simulink model "blance_robot"  (R2024a)
settings: Solver=VariableStepAuto  StartTime=0.0  StopTime=20  RelTol=1e-3
values from neighbouring files (symbols this model uses):
  K_cons = [-4.92635870386 -6.18040077772 -1.81074270733 -1.19207999822 -32.1009473092 -3.5760389828 4.18688097447 0.16514939939 0.944125254207 0.571537384386 -4.92635870394 -6.18040077751 ... (240 elements, 40x6)]    [K_cons.mat]    (also in k_calc.m = zeros(40,6))
  X = [x1, x2, x1sq, x2sq, x1x2]    [k_calc.m]
undefined symbols (not defined in the file or in its folder): Y, Z
libraries: sm_lib x58, nesl_utility x18, slpidlib x2
(part 1 of 3)
settings Model: Creator=zhuho  LastModifiedBy=zhuho

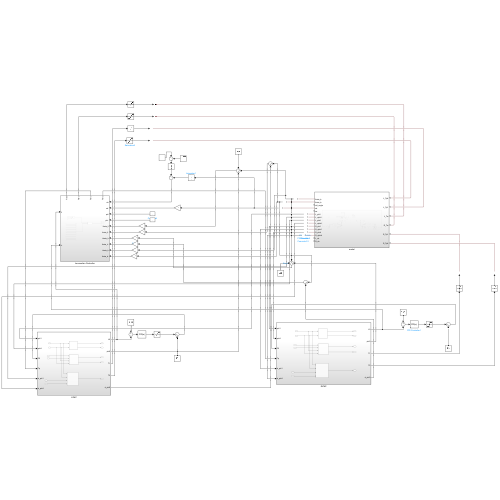
[thumbnail: Simulink's stored preview of the top-level diagram]
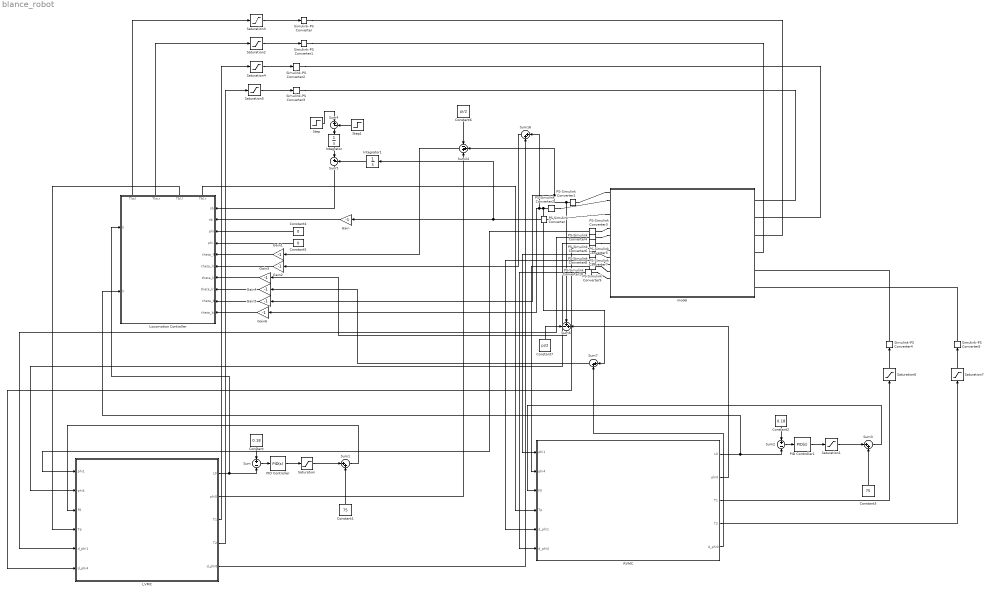
== system blance_robot ==
  Constant : Constant  Value=0.18
  Constant1 : Constant  Value=75
  Constant2 : Constant  Value=0.18
  Constant3 : Constant  Value=75
  Constant4 : Constant  Value=0
  Constant5 : Constant  Value=0
  Constant6 : Constant  Value=pi/2
  Constant7 : Constant  Value=pi/2
  Gain{,1..6} (7 alike) : Gain  Gain=-1
  Integrator : Integrator
  Integrator1 : Integrator
  LVMC : Subsystem
  Locomotion Controller : Subsystem
      settings: PortSchema="{\"entries\":[{\"content\":{\"sides\":[{\"content\":{\"connectorIds\":[\"In1\",\"In2\"]},\"type\":\"ConnectorPlacement.EquallySpacedRectSide\",\"uuid\":\"9f335f1a-920c-489c-ab23-b2605db4f7eb\"},{\"content\":{\"connectorIds\":[\"In3\",\"In4\",\"In5\",\"In6\",\"In7\",\"In8\",\"In9\",\"In10\",\"In11\",\"In12\"],\"side\":\"RIGHT\"},\"type\":\"ConnectorPlacement.EquallySpacedRectSide\",\"uuid\":\"244eb674-a427-495d-a4b5-69ad08e1900d\"},{\"content\":{\"connectorIds\":[\"Out1\",\"Out2\",\"Out3\",\"Out4\"],\"side\":\"TOP\"},\"type\":\"ConnectorPlacement.EquallySpacedRectSide\",\"uuid\":\"a2322f66-0ec6-4fc3-82d4-b6858da1a4af\"}]},\"type\":\"ConnectorPlacement.EquallySpacedConnector\",\"uuid\":\"7ddcb355-7f50-43e9-8496-f4eccb1abc77\"}],\"packageUris\":[\"http://schema.mathworks.com/mf0/Connector/R2020b\"],\"version\":\"1.0\"}"
  PID Controller : slpidlib/PID Controller  Controller=PID  Form=Parallel  TimeDomain=Continuous-time  UseExternalTs=off  SampleTime=-1  IntegratorMethod=Forward Euler  FilterMethod=Forward Euler  ControllerParametersSource=internal  P=500  I=0  UseKiTs=off  D=200  UseExternalDerivativeSource=off  N=100  UseFilter=on  TunerSelectOption=Transfer Function Based (PID Tuner App)  InitialConditionSource=internal  InitialConditionForIntegrator=0  InitialConditionForFilter=0  DifferentiatorICPrevScaledInput=0  ExternalReset=none  TrackingMode=off  Kt=1  LimitOutput=off  SatLimitsSource=internal  UpperSaturationLimit=inf  LowerSaturationLimit=-inf  LinearizeAsGain=on  AntiWindupMode=none  Kb=1  LimitIntegrator=off  UpperIntegratorSaturationLimit=inf  LowerIntegratorSaturationLimit=-inf  POutMin=[]  POutMax=[]  IOutMin=[]  IOutMax=[]  DOutMin=[]  DOutMax=[]  NOutMin=[]  NOutMax=[]  SumOutMin=[]  SumOutMax=[]  SaturationOutMin=[]  SaturationOutMax=[]  PParamMin=[]  PParamMax=[]  IParamMin=[]  IParamMax=[]  DParamMin=[]  DParamMax=[]  NParamMin=[]  NParamMax=[]  KbParamMin=[]  KbParamMax=[]  KtParamMin=[]  KtParamMax=[]  KbOutMin=[]  KbOutMax=[]  KtOutMin=[]  KtOutMax=[]  IntegratorOutMin=[]  IntegratorOutMax=[]  FilterOutMin=[]  FilterOutMax=[]  SumI1OutMin=[]  SumI1OutMax=[]  SumI2OutMin=[]  SumI2OutMax=[]  SumI3OutMin=[]  SumI3OutMax=[]  SumI4OutMin=[]  SumI4OutMax=[]  SumDOutMin=[]  SumDOutMax=[]  DifferentiatorOutMin=[]  DifferentiatorOutMax=[]  FilterDiffOutCoefMin=[]  FilterDiffOutCoefMax=[]  ReciprocalOutMin=[]  ReciprocalOutMax=[]  SumDenOutMin=[]  SumDenOutMax=[]  SumNumOutMin=[]  SumNumOutMax=[]  DivideOutMin=[]  DivideOutMax=[]  UdiffTsProdOutMin=[]  UdiffTsProdOutMax=[]  NTsProdOutMin=[]  NTsProdOutMax=[]  UintegralTsProdOutMin=[]  UintegralTsProdOutMax=[]  UngainTsProdOutMin=[]  UngainTsProdOutMax=[]  ClampingZeroOutDataTypeStr=Inherit: Inherit via back propagation  ClampingZeroOutMin=[]  ClampingZeroOutMax=[]  FilterDenConstantOutDataTypeStr=Inherit: Inherit via back propagation  FilterDenConstantOutMin=[]  FilterDenConstantOutMax=[]  PCopyOutDataTypeStr=Inherit: Inherit via back propagation  PCopyOutMin=[]  PCopyOutMax=[]  NCopyOutDataTypeStr=Inherit: Inherit via back propagation  NCopyOutMin=[]  NCopyOutMax=[]  IntegratorContinuousStateAttributes=''  IntegratorStateMustResolveToSignalObject=off  IntegratorRTWStateStorageClass=Auto  FilterContinuousStateAttributes=''  FilterStateMustResolveToSignalObject=off  FilterRTWStateStorageClass=Auto  ParallelPVariant=InternalParameters  IdealPVariant=Disabled  IVariant=InternalParameters  DVariant=InternalParameters  IntegratorVariant=Continuous  SatVariant=Disabled  AWVariant=Passthrough  PCopyVariant=Disabled  TRVariant=Disabled  FdbkBlocksVariant=Forward  IdealPFdbkVariant=Disabled  SatFdbkVariant=Disabled  DerivativeFilterVariant=ContFilter  NVariant=InternalParameters  NCopyVariant=Disabled  FilterICVariant=InternalICsFilter  IntegratorICVariant=InternalICs  ExternalResetVariant=Disabled  TRSumVariant=Passthrough  SumFdbkVariant=Disabled  SumVariant=Sum_PID  TsampFilterVariant=InternalTs  TsampNgainVariant=Passthrough  TsampIntegralVariant=Disabled_SignalSpec  ExternalSaturationOutDataTypeStr=Inherit: Same as second input  DerivativeSourceVariant=ErrorSignal
  PID Controller1 : slpidlib/PID Controller  Controller=PID  Form=Parallel  TimeDomain=Continuous-time  UseExternalTs=off  SampleTime=-1  IntegratorMethod=Forward Euler  FilterMethod=Forward Euler  ControllerParametersSource=internal  P=500  I=0  UseKiTs=off  D=200  UseExternalDerivativeSource=off  N=100  UseFilter=on  TunerSelectOption=Transfer Function Based (PID Tuner App)  InitialConditionSource=internal  InitialConditionForIntegrator=0  InitialConditionForFilter=0  DifferentiatorICPrevScaledInput=0  ExternalReset=none  TrackingMode=off  Kt=1  LimitOutput=off  SatLimitsSource=internal  UpperSaturationLimit=inf  LowerSaturationLimit=-inf  LinearizeAsGain=on  AntiWindupMode=none  Kb=1  LimitIntegrator=off  UpperIntegratorSaturationLimit=inf  LowerIntegratorSaturationLimit=-inf  POutMin=[]  POutMax=[]  IOutMin=[]  IOutMax=[]  DOutMin=[]  DOutMax=[]  NOutMin=[]  NOutMax=[]  SumOutMin=[]  SumOutMax=[]  SaturationOutMin=[]  SaturationOutMax=[]  PParamMin=[]  PParamMax=[]  IParamMin=[]  IParamMax=[]  DParamMin=[]  DParamMax=[]  NParamMin=[]  NParamMax=[]  KbParamMin=[]  KbParamMax=[]  KtParamMin=[]  KtParamMax=[]  KbOutMin=[]  KbOutMax=[]  KtOutMin=[]  KtOutMax=[]  IntegratorOutMin=[]  IntegratorOutMax=[]  FilterOutMin=[]  FilterOutMax=[]  SumI1OutMin=[]  SumI1OutMax=[]  SumI2OutMin=[]  SumI2OutMax=[]  SumI3OutMin=[]  SumI3OutMax=[]  SumI4OutMin=[]  SumI4OutMax=[]  SumDOutMin=[]  SumDOutMax=[]  DifferentiatorOutMin=[]  DifferentiatorOutMax=[]  FilterDiffOutCoefMin=[]  FilterDiffOutCoefMax=[]  ReciprocalOutMin=[]  ReciprocalOutMax=[]  SumDenOutMin=[]  SumDenOutMax=[]  SumNumOutMin=[]  SumNumOutMax=[]  DivideOutMin=[]  DivideOutMax=[]  UdiffTsProdOutMin=[]  UdiffTsProdOutMax=[]  NTsProdOutMin=[]  NTsProdOutMax=[]  UintegralTsProdOutMin=[]  UintegralTsProdOutMax=[]  UngainTsProdOutMin=[]  UngainTsProdOutMax=[]  ClampingZeroOutDataTypeStr=Inherit: Inherit via back propagation  ClampingZeroOutMin=[]  ClampingZeroOutMax=[]  FilterDenConstantOutDataTypeStr=Inherit: Inherit via back propagation  FilterDenConstantOutMin=[]  FilterDenConstantOutMax=[]  PCopyOutDataTypeStr=Inherit: Inherit via back propagation  PCopyOutMin=[]  PCopyOutMax=[]  NCopyOutDataTypeStr=Inherit: Inherit via back propagation  NCopyOutMin=[]  NCopyOutMax=[]  IntegratorContinuousStateAttributes=''  IntegratorStateMustResolveToSignalObject=off  IntegratorRTWStateStorageClass=Auto  FilterContinuousStateAttributes=''  FilterStateMustResolveToSignalObject=off  FilterRTWStateStorageClass=Auto  ParallelPVariant=InternalParameters  IdealPVariant=Disabled  IVariant=InternalParameters  DVariant=InternalParameters  IntegratorVariant=Continuous  SatVariant=Disabled  AWVariant=Passthrough  PCopyVariant=Disabled  TRVariant=Disabled  FdbkBlocksVariant=Forward  IdealPFdbkVariant=Disabled  SatFdbkVariant=Disabled  DerivativeFilterVariant=ContFilter  NVariant=InternalParameters  NCopyVariant=Disabled  FilterICVariant=InternalICsFilter  IntegratorICVariant=InternalICs  ExternalResetVariant=Disabled  TRSumVariant=Passthrough  SumFdbkVariant=Disabled  SumVariant=Sum_PID  TsampFilterVariant=InternalTs  TsampNgainVariant=Passthrough  TsampIntegralVariant=Disabled_SignalSpec  ExternalSaturationOutDataTypeStr=Inherit: Same as second input  DerivativeSourceVariant=ErrorSignal
  PS-Simulink Converter{,1..10} (11 alike) : nesl_utility/PS-Simulink Converter  PhysicalDomain=network_engine_domain  SubClassName=ps_output  LeftPortType=input  RightPortType=output  PseudoPeriodic=off  Frequencies=[]  VectorFormat=inherit  Unit=inherit  AffineConversion=off
  RVMC : Subsystem
  Saturation : Saturate  UpperLimit=9  LowerLimit=-9
  Saturation1 : Saturate  UpperLimit=9  LowerLimit=-9
  Saturation{2..7} (6 alike) : Saturate  UpperLimit=10  LowerLimit=-10
  Simulink-PS Converter{,1..5} (6 alike) : nesl_utility/Simulink-PS Converter  PhysicalDomain=network_engine_domain  SubClassName=ps_input  LeftPortType=input  RightPortType=output  PseudoPeriodic=off  Frequencies=[]  NoiseDistribution=none  NoiseParameters=[]  Unit=1  AffineConversion=off  FilteringAndDerivatives=provide  SimscapeFilterOrder=1  InputFilterTimeConstant=0.001  UdotUserProvided=0
  Step : Step  Time=0.8  After=2.5  SampleTime=0
  Step1 : Step  Time=5  After=2.5  SampleTime=0
  Sum : Sum  Inputs=+|-
  Sum{1,3,7,16} (4 alike) : Sum  Inputs=|++
  Sum2 : Sum  Inputs=+|-
  Sum24 : Sum  Inputs=-++
  Sum4 : Sum  Inputs=|+-
  Sum5 : Sum  Inputs=|+-
  Sum6 : Sum  Inputs=-++
  model : Subsystem
  wires:
  Constant/1 -> Sum/1
  Sum/1 -> PID Controller/1
  PID Controller/1 -> Saturation/1
  Constant1/1 -> Sum1/2
  Saturation/1 -> Sum1/1
  Sum1/1 -> LVMC/3(F0)
  Locomotion Controller/3(Tbl,l) -> LVMC/4(Tp)
  Locomotion Controller/4(Tbl,r) -> RVMC/4(Tp)
  Constant2/1 -> Sum2/1
  Sum2/1 -> PID Controller1/1
  PID Controller1/1 -> Saturation1/1
  Constant3/1 -> Sum3/2
  Saturation1/1 -> Sum3/1
  Sum3/1 -> RVMC/3(F0)
  LVMC/1(L0) -> Locomotion Controller/1(ll), Sum/2
  RVMC/1(L0) -> Locomotion Controller/2(lr), Sum2/2
  Locomotion Controller/1(Tlw,l) -> Saturation3/1
  Locomotion Controller/2(Tlw,r) -> Saturation2/1
  Saturation2/1 -> Simulink-PS Converter1/1
  Saturation3/1 -> Simulink-PS Converter/1
  LVMC/4(T2) -> Saturation5/1
  LVMC/3(T1) -> Saturation4/1
  Saturation4/1 -> Simulink-PS Converter2/1
  Saturation5/1 -> Simulink-PS Converter3/1
  RVMC/3(T1) -> Saturation6/1
  Saturation6/1 -> Simulink-PS Converter4/1
  RVMC/4(T2) -> Saturation7/1
  Saturation7/1 -> Simulink-PS Converter5/1
  PS-Simulink Converter/1 -> Integrator1/1, Gain/1
  Gain/1 -> Locomotion Controller/4(sb.)
  Step/1 -> Sum4/1
  Step1/1 -> Sum4/2
  Sum4/1 -> Integrator/1
  Integrator/1 -> Sum5/1
  Sum5/1 -> Locomotion Controller/3(sb)
  Integrator1/1 -> Sum5/2
  Constant4/1 -> Locomotion Controller/5(phi)
  Constant5/1 -> Locomotion Controller/6(phi.)
  Constant6/1 -> Sum24/1
  Sum24/1 -> Gain1/1
  LVMC/2(phi0) -> Sum24/3
  PS-Simulink Converter1/1 -> Gain5/1, Sum24/2, Sum6/2
  Gain1/1 -> Locomotion Controller/7(theta_ll)
  PS-Simulink Converter2/1 -> Sum7/1, Gain6/1, Sum16/1
  LVMC/5(d_phi0) -> Sum16/2
  Sum16/1 -> Gain2/1
  Gain2/1 -> Locomotion Controller/8(theta_ll.)
  Constant7/1 -> Sum6/1
  RVMC/2(phi0) -> Sum6/3
  Sum6/1 -> Gain3/1
  RVMC/5(d_phi0) -> Sum7/2
  Sum7/1 -> Gain4/1
  Gain3/1 -> Locomotion Controller/9(theta_lr)
  Gain4/1 -> Locomotion Controller/10(theta_lr.)
  Gain5/1 -> Locomotion Controller/11(theta_b)
  Gain6/1 -> Locomotion Controller/12(theta_b.)
  PS-Simulink Converter3/1 -> LVMC/1(phi1)
  PS-Simulink Converter4/1 -> LVMC/5(d_phi1)
  PS-Simulink Converter5/1 -> LVMC/2(phi4)
  PS-Simulink Converter6/1 -> LVMC/6(d_phi4)
  PS-Simulink Converter7/1 -> RVMC/1(phi1)
  PS-Simulink Converter9/1 -> RVMC/2(phi4)
  PS-Simulink Converter8/1 -> RVMC/5(d_phi1)
  PS-Simulink Converter10/1 -> RVMC/6(d_phi4)
  connections:
  model/RConn4 -- PS-Simulink Converter/LConn1
  Simulink-PS Converter/RConn1 -- model/LConn3
  Simulink-PS Converter1/RConn1 -- model/LConn4
  Simulink-PS Converter2/RConn1 -- model/LConn2
  Simulink-PS Converter3/RConn1 -- model/LConn1
  Simulink-PS Converter4/RConn1 -- model/LConn5
  Simulink-PS Converter5/RConn1 -- model/LConn6
  model/RConn1 -- PS-Simulink Converter1/LConn1
  PS-Simulink Converter2/LConn1 -- model/RConn2
  PS-Simulink Converter3/LConn1 -- model/RConn6
  PS-Simulink Converter4/LConn1 -- model/RConn7
  PS-Simulink Converter5/LConn1 -- model/RConn8
  PS-Simulink Converter6/LConn1 -- model/RConn9
  PS-Simulink Converter7/LConn1 -- model/RConn10
  PS-Simulink Converter8/LConn1 -- model/RConn11
  PS-Simulink Converter9/LConn1 -- model/RConn12
  PS-Simulink Converter10/LConn1 -- model/RConn13

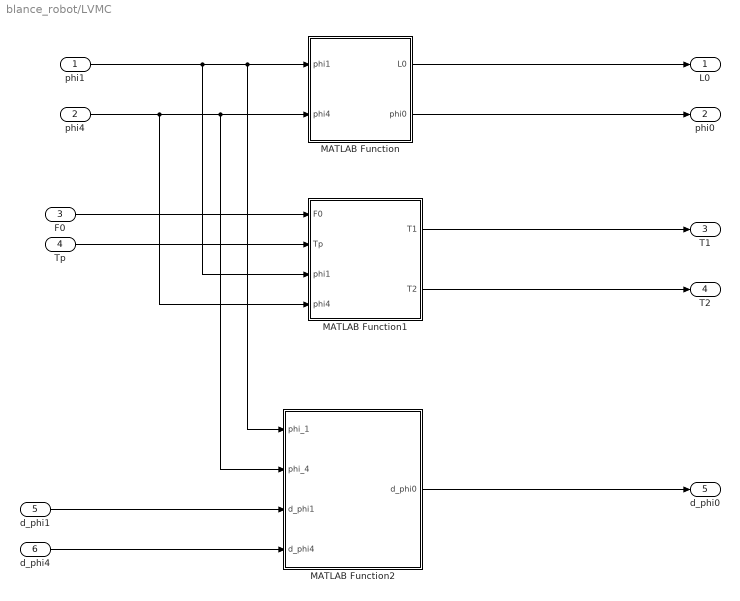
== system blance_robot/LVMC ==
  phi1 : Inport
  phi4 : Inport  Port=2
  F0 : Inport  Port=3
  Tp : Inport  Port=4
  d_phi1 : Inport  Port=5
  d_phi4 : Inport  Port=6
  MATLAB Function : MATLAB Function  TreatAsAtomicUnit=on
  MATLAB Function1 : MATLAB Function  TreatAsAtomicUnit=on
  MATLAB Function2 : MATLAB Function  TreatAsAtomicUnit=on
  L0 : Outport
  phi0 : Outport  Port=2
  T1 : Outport  Port=3
  T2 : Outport  Port=4
  d_phi0 : Outport  Port=5
  wires:
  phi1/1 -> MATLAB Function1/3(phi1), MATLAB Function2/1(phi_1), MATLAB Function/1(phi1)
  phi4/1 -> MATLAB Function1/4(phi4), MATLAB Function2/2(phi_4), MATLAB Function/2(phi4)
  F0/1 -> MATLAB Function1/1(F0)
  Tp/1 -> MATLAB Function1/2(Tp)
  d_phi1/1 -> MATLAB Function2/3(d_phi1)
  d_phi4/1 -> MATLAB Function2/4(d_phi4)
  MATLAB Function/1(L0) -> L0/1
  MATLAB Function/2(phi0) -> phi0/1
  MATLAB Function1/1(T1) -> T1/1
  MATLAB Function1/2(T2) -> T2/1
  MATLAB Function2/1(d_phi0) -> d_phi0/1

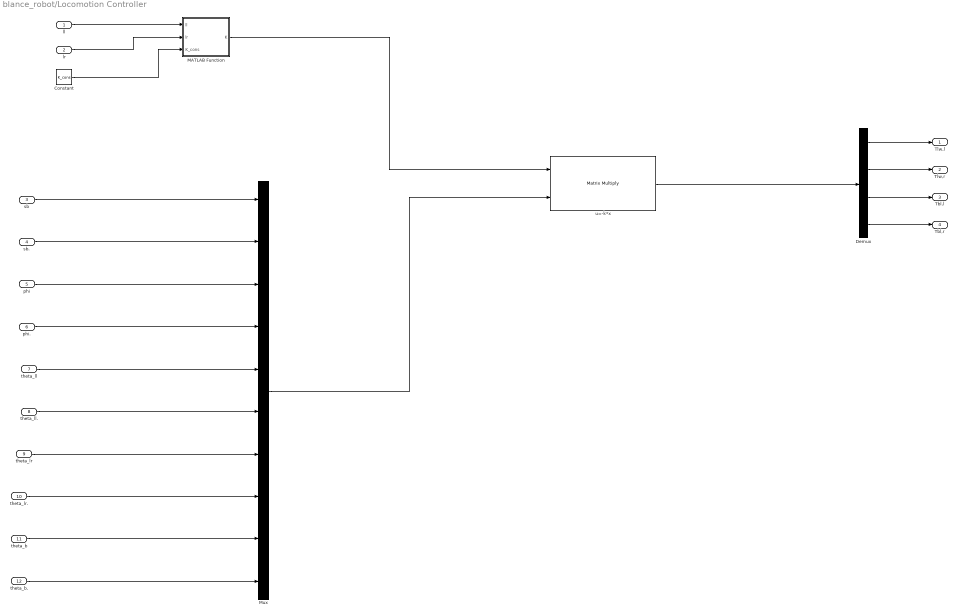
== system blance_robot/Locomotion Controller ==
  ll : Inport
  lr : Inport  Port=2
  sb : Inport  Port=3
  sb. : Inport  Port=4
  phi : Inport  Port=5
  phi. : Inport  Port=6
  theta_ll : Inport  Port=7
  theta_ll. : Inport  Port=8
  theta_lr : Inport  Port=9
  theta_lr. : Inport  Port=10
  theta_b : Inport  Port=11
  theta_b. : Inport  Port=12
  Constant : Constant  Value=K_cons
  Demux : Demux
  MATLAB Function : MATLAB Function  TreatAsAtomicUnit=on
  Mux : Mux  Inputs=10
  u=-k*x : Product  Multiplication=Matrix(*)
  Tlw,l : Outport
  Tlw,r : Outport  Port=2
  Tbl,l : Outport  Port=3
  Tbl,r : Outport  Port=4
  wires:
  ll/1 -> MATLAB Function/1(ll)
  lr/1 -> MATLAB Function/2(lr)
  Constant/1 -> MATLAB Function/3(K_cons)
  sb/1 -> Mux/1
  sb./1 -> Mux/2
  phi/1 -> Mux/3
  phi./1 -> Mux/4
  theta_ll/1 -> Mux/5
  theta_ll./1 -> Mux/6
  theta_lr/1 -> Mux/7
  theta_lr./1 -> Mux/8
  theta_b/1 -> Mux/9
  theta_b./1 -> Mux/10
  MATLAB Function/1(K) -> u=-k*x/1
  Mux/1 -> u=-k*x/2
  u=-k*x/1 -> Demux/1
  Demux/1 -> Tlw,l/1
  Demux/2 -> Tlw,r/1
  Demux/3 -> Tbl,l/1
  Demux/4 -> Tbl,r/1

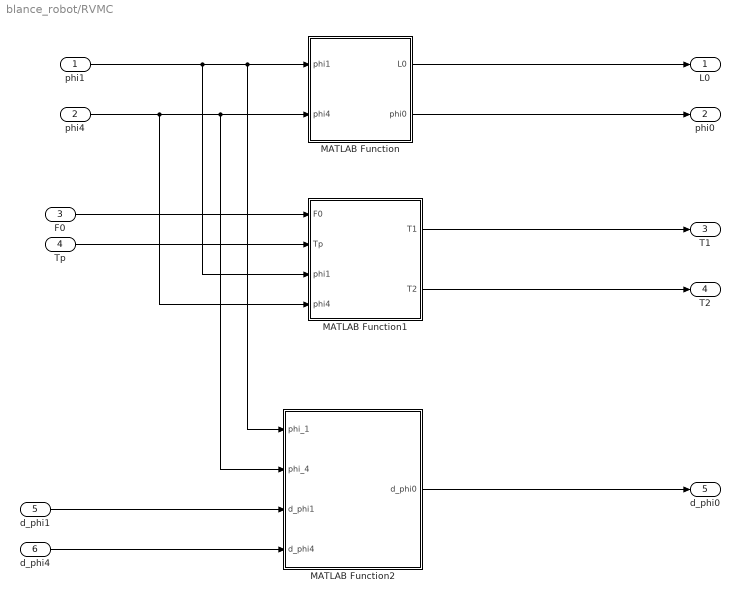
== system blance_robot/RVMC ==
  phi1 : Inport
  phi4 : Inport  Port=2
  F0 : Inport  Port=3
  Tp : Inport  Port=4
  d_phi1 : Inport  Port=5
  d_phi4 : Inport  Port=6
  MATLAB Function : MATLAB Function  TreatAsAtomicUnit=on
  MATLAB Function1 : MATLAB Function  TreatAsAtomicUnit=on
  MATLAB Function2 : MATLAB Function  TreatAsAtomicUnit=on
  L0 : Outport
  phi0 : Outport  Port=2
  T1 : Outport  Port=3
  T2 : Outport  Port=4
  d_phi0 : Outport  Port=5
  wires:
  phi1/1 -> MATLAB Function1/3(phi1), MATLAB Function2/1(phi_1), MATLAB Function/1(phi1)
  phi4/1 -> MATLAB Function1/4(phi4), MATLAB Function2/2(phi_4), MATLAB Function/2(phi4)
  F0/1 -> MATLAB Function1/1(F0)
  Tp/1 -> MATLAB Function1/2(Tp)
  d_phi1/1 -> MATLAB Function2/3(d_phi1)
  d_phi4/1 -> MATLAB Function2/4(d_phi4)
  MATLAB Function/1(L0) -> L0/1
  MATLAB Function/2(phi0) -> phi0/1
  MATLAB Function1/1(T1) -> T1/1
  MATLAB Function1/2(T2) -> T2/1
  MATLAB Function2/1(d_phi0) -> d_phi0/1
